simulink model "DebounceAlgorithm"  (R2021b)
settings: Solver=VariableStepAuto  StartTime=0.0  StopTime=10.0  RelTol=1e-3
values from neighbouring files (symbols this model uses):
  Trsh = 1000    [DebounceParams.m]
  Ts = 0.0001    [DebounceParams.m]
settings Model: Creator=win  LastModifiedBy=win

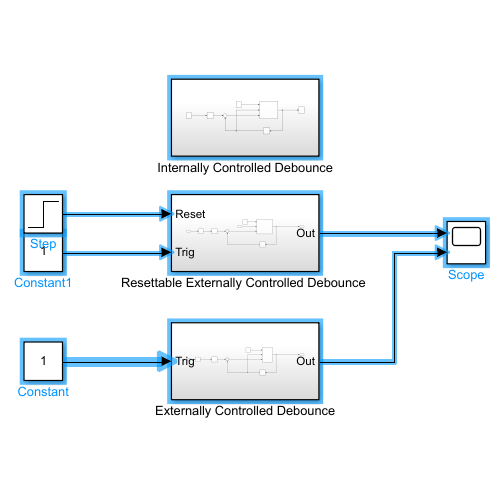
[thumbnail: Simulink's stored preview of the top-level diagram]
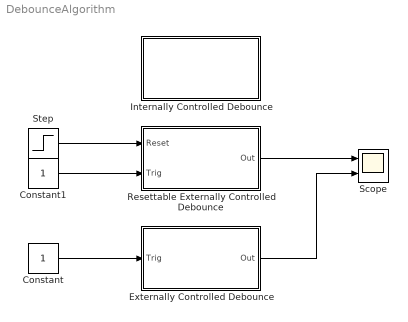
== system DebounceAlgorithm ==
  Constant : Constant
  Constant1 : Constant
  Externally Controlled Debounce : Subsystem
  Internally Controlled Debounce : Subsystem
  "Resettable Externally Controlled Debounce " : Subsystem
  Scope : Scope  NumInputPorts=2
  Step : Step  SampleTime=0
  wires:
  Step/1 -> "Resettable Externally Controlled Debounce "/1(Reset)
  Externally Controlled Debounce/1(Out) -> Scope/2
  Constant1/1 -> "Resettable Externally Controlled Debounce "/2(Trig)
  "Resettable Externally Controlled Debounce "/1(Out) -> Scope/1
  Constant/1 -> Externally Controlled Debounce/1(Trig)

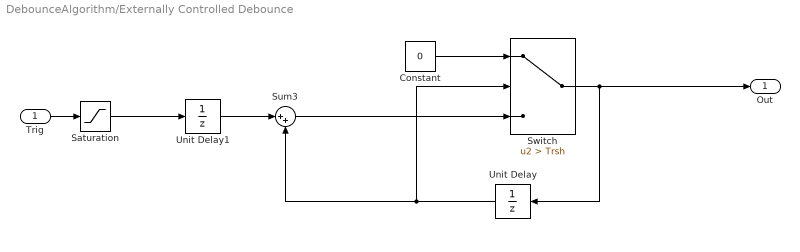
== system DebounceAlgorithm/Externally Controlled Debounce ==
  Trig : Inport
  Constant : Constant  Value=0
  Saturation : Saturate  UpperLimit=1  LowerLimit=0
  Sum3 : Sum  Inputs=|++
  Switch : Switch  Criteria=u2 > Threshold  Threshold=Trsh
  Unit Delay : UnitDelay  SampleTime=Ts  HasFrameUpgradeWarning=on
  Unit Delay1 : UnitDelay  SampleTime=Ts  HasFrameUpgradeWarning=on
  Out : Outport
  wires:
  Saturation/1 -> Unit Delay1/1
  Unit Delay/1 -> Switch/2, Sum3/2
  Trig/1 -> Saturation/1
  Constant/1 -> Switch/1
  Switch/1 -> Unit Delay/1, Out/1
  Sum3/1 -> Switch/3
  Unit Delay1/1 -> Sum3/1

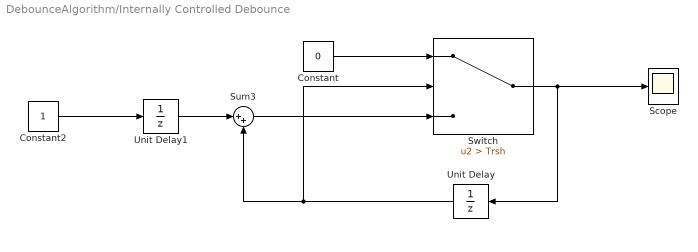
== system DebounceAlgorithm/Internally Controlled Debounce ==
  Constant : Constant  Value=0
  Constant2 : Constant
  Scope : Scope
  Sum3 : Sum  Inputs=|++
  Switch : Switch  Criteria=u2 > Threshold  Threshold=Trsh
  Unit Delay : UnitDelay  SampleTime=Ts  HasFrameUpgradeWarning=on
  Unit Delay1 : UnitDelay  SampleTime=Ts  HasFrameUpgradeWarning=on
  wires:
  Unit Delay/1 -> Switch/2, Sum3/2
  Constant2/1 -> Unit Delay1/1
  Constant/1 -> Switch/1
  Switch/1 -> Unit Delay/1, Scope/1
  Sum3/1 -> Switch/3
  Unit Delay1/1 -> Sum3/1

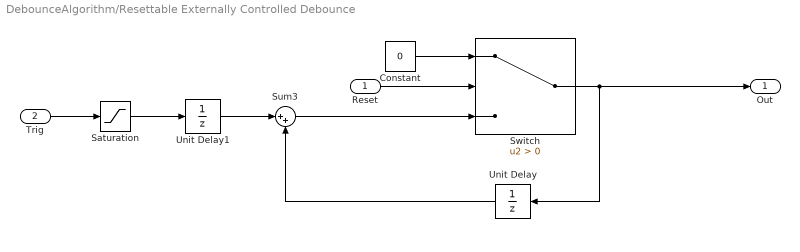
== system DebounceAlgorithm/Resettable Externally Controlled Debounce  ==
  Reset : Inport
  Trig : Inport  Port=2
  Constant : Constant  Value=0
  Saturation : Saturate  UpperLimit=1  LowerLimit=0
  Sum3 : Sum  Inputs=|++
  Switch : Switch  Criteria=u2 > Threshold
  Unit Delay : UnitDelay  SampleTime=Ts  HasFrameUpgradeWarning=on
  Unit Delay1 : UnitDelay  SampleTime=Ts  HasFrameUpgradeWarning=on
  Out : Outport
  wires:
  Unit Delay1/1 -> Sum3/1
  Sum3/1 -> Switch/3
  Switch/1 -> Out/1, Unit Delay/1
  Constant/1 -> Switch/1
  Trig/1 -> Saturation/1
  Unit Delay/1 -> Sum3/2
  Saturation/1 -> Unit Delay1/1
  Reset/1 -> Switch/2
